simulink model "Waehrungsmodelle"  (R2014a)
settings: Solver=ode1  StartTime=0.0  StopTime=100  FixedStep=1  MaxStep=1  MinStep=1  RelTol=1e-3
(part 2 of 18)

== matlab function Waehrungsmodelle/Währungssystem2/Notenbank/MATLAB Function ==
  data: Gesamtkredite input; LeitzinsOut output; MindestreservesatzOut output; MaximaleNotenbankGeldmengeOut output; Arbeitslosenquote input; Inflation input; Wirtschaftswachtsum input
function [LeitzinsOut, MindestreservesatzOut, MaximaleNotenbankGeldmengeOut] = ...
    Notenbank(Gesamtkredite, Arbeitslosenquote, Inflation, Wirtschaftswachtsum)
%# Submodul zur Berechnung der Notenbankprozesse

% Leitzins der Notenbank => 0.03
persistent Leitzins;

% Mindestreservesatz => 0.01
persistent Mindestreservesatz;    

% Maximale Geldmenge, welche von der Notenbank vergeben werden kann
persistent MaximaleNotenbankGeldmenge;   

% festgelegter Geldmengenwachstum => 0.05
% Dieser Wert ist bei gedeckten Währungssystemen notwendig, da hiermit die
% Geldmenge mit dem Gesamtwert des Deckungswerts mitwachsen kann
Geldmengenwachstum = 0.05;

% gewünschte Inflation => 0.02
Inflationsziel = 0.02;

% Inflationstoleranz => 0.02
Inflationstoleranz = 0.02;

% Arbeitslosentoleranzquote => 0.08
Arbeitslosentoleranzquote = 0.08;

% Änderung des Leitzins
Leitzinsaenderung = 0;

    if isempty(Leitzins)
       Leitzins = 0.03;
    end  
    if isempty(Mindestreservesatz)
       Mindestreservesatz = 0.01;
    end  
    if isempty(MaximaleNotenbankGeldmenge)
       MaximaleNotenbankGeldmenge =  1000;
    end       
    
    % Pürfen, ob ein erlaubter Geldmengenwachstum sinnvoll ist
    if Gesamtkredite > MaximaleNotenbankGeldmenge * 0.9
        MaximaleNotenbankGeldmenge = MaximaleNotenbankGeldmenge * (1 + Geldmengenwachstum);
    end
    
    % Wenn das Wirtschaftswachtsum zu gering ist, wird der Leitzins gesenkt
    if Wirtschaftswachtsum < Leitzins
        Leitzinsaenderung = -0.001;
    else
        Leitzinsaenderung = 0.001;
    end
    
    % Wenn die Arbeitslosigkeit unter der Arbeitslosentoleranzquote ist, wird kann der Leitzins erhöht
    % sonst wird der Leitzins in Abhängigkeit der Arbeitslosenquote gesenkt
    Leitzinsaenderung = Leitzinsaenderung + max(-0.01,0.1 * (Arbeitslosentoleranzquote - Arbeitslosenquote) + 0.001);
    
    % Inflation mit dem Leitzins an die Zielinflation anpassen
    Leitzinsaenderung = Leitzinsaenderung + 0.01 * (Inflation - (Inflationsziel + Inflationstoleranz));
        
    if Leitzins < 0.01 && Leitzinsaenderung < -0.001
        Leitzins = Leitzins - 0.001;
    else        
        Leitzins = Leitzins + Leitzinsaenderung;
    end
    
LeitzinsOut = Leitzins;
MindestreservesatzOut = Mindestreservesatz;
MaximaleNotenbankGeldmengeOut = MaximaleNotenbankGeldmenge;

== matlab function Waehrungsmodelle/Währungssystem2/Unternehmen/MATLAB Function ==
  data: Inflation output; Rohstoffbedarf output; ArbeitsplaetzeUnternehmen output; GueterangebotInland output; ArbeitslohnOut output; Erwerbsfaehige input; BenoetigterArbeitsbedarfUnternehmen output; GueterpreisOut output; NeueKreditvergabeUnternehmen input; KreditrueckzahlungUnternehmen input; SteuernUnternehmen output; RessourcenAbgabeSteuer output; KreditbedarfInland output; Rohstoffe input; GueterkonsumInland input; GueterkonsumAusland input; RessourcenAbgabeSteuersatz input; KreditZinssatzInland input; KreditZinssatzAusland input; Steuersatz input; KreditbedarfAusland output; TechnischeVerbesserungRationalitaetOut output; TechnischeVerbesserungRessourcenOut output; Wirtschaftswachstum output; GueterangebotAusland output; NeueKreditvergabeUnternehmenAusland input; KreditrueckzahlungUnternehmenAusland input
function [Inflation, Rohstoffbedarf, ArbeitsplaetzeUnternehmen, GueterangebotInland, ...
            ArbeitslohnOut, BenoetigterArbeitsbedarfUnternehmen, GueterpreisOut, ...
            SteuernUnternehmen, RessourcenAbgabeSteuer, KreditbedarfInland, KreditbedarfAusland,  ...
            TechnischeVerbesserungRationalitaetOut, TechnischeVerbesserungRessourcenOut, ...
            Wirtschaftswachstum, GueterangebotAusland] = ...
   Unternehmen(Erwerbsfaehige, NeueKreditvergabeUnternehmen, KreditrueckzahlungUnternehmen, ...
            Rohstoffe, GueterkonsumInland, GueterkonsumAusland, RessourcenAbgabeSteuersatz, ...
            KreditZinssatzInland, KreditZinssatzAusland, Steuersatz, ...
            NeueKreditvergabeUnternehmenAusland, KreditrueckzahlungUnternehmenAusland)
        %# Submodul zur Berechnung der Prozessabläufe in Beziehung mit den Unternehmen

% Arbeitslohn
persistent Arbeitslohn;          
        
% Geldbestand
persistent Geldbestand;  
        
% Rohstoffbestand
persistent Rohstoffbestand;   
        
% produzierter Güterbestand
persistent Gueterbestand;   

% Preis zu dem das produzierte Gut verkauft wird
persistent Gueterpreis;  

% technische Effizienzverbesserung bzgl. der Rationalisierung der Arbeiter
persistent TechnischeVerbesserungRationalitaet;   

% technische Effizienzverbesserung bzgl. der Ressourcenverwendung
persistent TechnischeVerbesserungRessourcen;

% Letzte Anzahl an Mitarbeitern
persistent LetzteArbeitsplaetzeUnternehmen;

% Umsatz / Einnahmen
persistent Einnahmen;

% alte Inflation
persistent InflationAlt;

% Geldbestand Initial
if isempty(Geldbestand)
   Geldbestand = 50;
end
% Arbeitslohn Initial
if isempty(Arbeitslohn)
   Arbeitslohn = 3.5;
end
% Rohstoffbestand Initial
if isempty(Rohstoffbestand)
   Rohstoffbestand = 50;
end
% Güterbestand Initial
if isempty(Gueterbestand)
   Gueterbestand = 50;
end 
% Güterpreis Initial
if isempty(Gueterpreis)
   Gueterpreis = 3;
end 
% technische Effizienzverbesserung Rationalisierung Initial
if isempty(TechnischeVerbesserungRessourcen)
   TechnischeVerbesserungRessourcen = 1;
end
% technische Effizienzverbesserung Ressourcenverwendung Initial
if isempty(TechnischeVerbesserungRationalitaet)
   TechnischeVerbesserungRationalitaet = 1;
end
% Umsatz / Einnahmen Initial
if isempty(Einnahmen)
   Einnahmen = 0;
end
if isempty(InflationAlt)
   InflationAlt = 0;
end
% Letzte Anzahl an Mitarbeitern
if isempty(LetzteArbeitsplaetzeUnternehmen)
   LetzteArbeitsplaetzeUnternehmen = 20;
end

% Steigerung der Effizienzen bei technischen Verbesserungen Rationalität
EffizienzsteigerungRationalitaet = 0.04;
% Steigerung der Effizienzen bei technischen Verbesserungen Ressourcen
EffizienzsteigerungRessourcen = 0.02;
% Kosten einer technischen Verbesserung
Verbesserungskosten = 20;
% Steigerung der Kosten bei technischen Verbesserungen
Verbesserungskostensteigerung = 0.2;
% Angestrebter Gewinn
AngestrebterGewinn = 0.1;
% Maximale Preissteierung
MaximalePreissteierung = 0.15;
% Speicherung des letzten Güterpreises
AlterGueterpreis = Gueterpreis;
% Speicherung der letzten Einnahmen
AlteEinnahmen = Einnahmen;
% Menge produzierter Güter pro Mitarbeiter
ProduzierteMengeProMitarbeiter = 1.2;
% Gehaltssteigerung bei Rationalisierung und Gewinn
Gehaltssteigerung = 0.05;
% angestrebter Gütervorrat
GewuenschterGuetervorrat = 200;
% angestrebter Geldbestand
GewuenschterGeldbestand = 200;
% Maximale Entlassungen in Prozent
MaximaleEntlassungsrate = 0.2;

    % vergebene Kredite
    Geldbestand = Geldbestand + NeueKreditvergabeUnternehmen + NeueKreditvergabeUnternehmenAusland;
    % Ratenzahlung der aktuelen Kredite
    Geldbestand = Geldbestand - KreditrueckzahlungUnternehmen + KreditrueckzahlungUnternehmenAusland;

    % Berechnung der Ressourcenangabe
    RessourcenAbgabeSteuer = max(0, RessourcenAbgabeSteuersatz) * Rohstoffe;
    Rohstoffbestand = Rohstoffbestand + Rohstoffe;
    
    % In- und Auslandskonsum summieren
    Gueterkonsum = GueterkonsumInland + GueterkonsumAusland;
    
    % Güterbestand nach den von abgenommene Güter der Haushalten bei 
    % der letzten Zeiteinheit 
    Gueterbestand = Gueterbestand - Gueterkonsum;
    
    % Berechnung der Einnahmen
    Einnahmen = Gueterkonsum * Gueterpreis;
    
    % Berechnung der zu produzierenden Gütermenge (mit 30% Reserve) wenn
    % der Bestand kleiner als 200% des Güterkonsums in einer Zeiteinheit
    % Dabei werden 50 Güter als Reserve in Bestand vorgehalten
    if Gueterbestand < Gueterkonsum * 2
        ProduzierndeGuetermenge = max(5, (1.3 * Gueterkonsum) - (Gueterbestand - GewuenschterGuetervorrat));  
    elseif Gueterbestand < GewuenschterGuetervorrat
        ProduzierndeGuetermenge = Gueterkonsum + (GewuenschterGuetervorrat - Gueterbestand);
    else
       ProduzierndeGuetermenge = max(5, Gueterkonsum / 2);      
    end
    
    % Produktiongüter pro Mitarbeiter in Abhängigkeit
    % der technischen Verbesserung (normal 2 Güter pro Mitarbeiter)
    ProduktionProMitarbeiter = (((1 + EffizienzsteigerungRationalitaet) ^ TechnischeVerbesserungRationalitaet) * ProduzierteMengeProMitarbeiter);
    
    % Ressourcen pro hergestelltes Gut in Abhängigkeit
    % der technischen Verbesserung (normal 1 Güter pro Ressource)    
    RessourcenProGut = (1 / (1 + EffizienzsteigerungRessourcen)) ^ TechnischeVerbesserungRessourcen;
    
    % Zur Berechnung der benötigten Arbeitskraft im nächsten Zeitabschnitt´
    BenoetigterArbeitsbedarfUnternehmen = floor(ProduzierndeGuetermenge / ProduktionProMitarbeiter) + 1;           
    
    % Berechnung der maximal erstellbaren Gütermenge
    MaximaleGueterherstellungErwerbstaetige = Erwerbsfaehige * ProduktionProMitarbeiter;
    MaximaleGueterherstellungRohstoffe = Rohstoffbestand / RessourcenProGut;    
    % Entweder ist die Herstellung durch die Nachfrage, den Arbeitskreaften
    % oder den Ressourcen beschränkt
    Gueterherstellung = min(ProduzierndeGuetermenge, min(MaximaleGueterherstellungErwerbstaetige, MaximaleGueterherstellungRohstoffe));
    Gueterherstellung = max(Gueterherstellung, 0);  
    
    % Berechnung der aktuellen Arbeitsplätze
    ArbeitsplaetzeUnternehmen = floor(Gueterherstellung / ProduktionProMitarbeiter)+1;
    
    % Berechnung der maximalen möglichen Entlassungen
    % Es können max. 20% der Mitarbeiter entlassen werden    
    if ArbeitsplaetzeUnternehmen < LetzteArbeitsplaetzeUnternehmen * (1-MaximaleEntlassungsrate)
        ArbeitsplaetzeUnternehmen = LetzteArbeitsplaetzeUnternehmen * (1-MaximaleEntlassungsrate);
        MaximaleGueterherstellungErwerbstaetige = ArbeitsplaetzeUnternehmen * ProduktionProMitarbeiter;
        Gueterherstellung = min(ProduzierndeGuetermenge, min(MaximaleGueterherstellungErwerbstaetige, MaximaleGueterherstellungRohstoffe));        
    end
    
    % Vergleich der Arbeitsnachfrage mit dem Arbeitsangebot
    ArbeitsangebotsNachfrageQuotient = ArbeitsplaetzeUnternehmen / Erwerbsfaehige;
    % Anpassung der Arbeitslöhne an das Angebot und die Nachfrage der
    % Arbeitsplaetze - max 3% Lohnsenkung oder Lohnsteigerung
    ArbeitsangebotsNachfrageQuotient= max(0.94,min(1.04,(ArbeitsangebotsNachfrageQuotient + 0.3)));
    Arbeitslohn = Arbeitslohn * ArbeitsangebotsNachfrageQuotient;
    
    % Berechnung der aktuell verbrauchten Ressourcen
    Rohstoffbestand = Rohstoffbestand - (floor(Gueterherstellung * RessourcenProGut)+1);
    
    % hergestellte Gütermenge
    Gueterbestand = Gueterbestand + Gueterherstellung;
    
    % Als Export-Angebot werden 30% der Güter vorgesehen
    GueterangebotAusland = Gueterbestand * 0.3;
    GueterangebotInland = Gueterbestand - GueterangebotAusland;          
    
    % Berechnung der Gehälter
    Gehaelter = ArbeitsplaetzeUnternehmen * Arbeitslohn;
    
    % Vorteil einer Investitionen-Rationalität berechnen
    InvestPruefungProduktionProMitarbeiter = (((1 + EffizienzsteigerungRationalitaet) ^ (TechnischeVerbesserungRationalitaet + 1)) * 2);
    InvestPruefungArbeitsplaetzeUnternehmen = floor(Gueterherstellung / InvestPruefungProduktionProMitarbeiter)+1;    
    InvesteinsparungRationalitaet = Arbeitslohn * (ArbeitsplaetzeUnternehmen - InvestPruefungArbeitsplaetzeUnternehmen);
    % Vorteil einer Investitionen-Ressourceneffizienz berechnen
    InvestPruefungRessourcenProGut = (1 / (1 + EffizienzsteigerungRessourcen)) ^ (TechnischeVerbesserungRessourcen + 1);
    InvestPruefungRessourcenbedarf = floor(Gueterherstellung * InvestPruefungRessourcenProGut)+1;    
    InvesteinsparungRessourcenbedarf = RessourcenAbgabeSteuersatz * ((Gueterherstellung * RessourcenProGut) - InvestPruefungRessourcenbedarf);    
    
    % Kosten für die nächste Investitionsstufe berechnen
    InvestkostenRationalitaet = Verbesserungskosten * (1 + Verbesserungskostensteigerung) ^ (TechnischeVerbesserungRationalitaet + 1);
    InvestkostenRessourcenEffizienz = Verbesserungskosten * (1 + Verbesserungskostensteigerung) ^ (TechnischeVerbesserungRessourcen + 1);
    
    % Prüfen, ob und welche Investition mehr Sinn macht
    % Das vorhandene Geld muss dabei doppelt so hoch sein, damit nicht mit
    % dem letzten Geld Investitionen durchgeführt werden
    Investition = 0;
    if (InvesteinsparungRationalitaet > InvesteinsparungRessourcenbedarf) && Geldbestand > InvestkostenRationalitaet*2 && InvesteinsparungRationalitaet > 0
        % Verbesserung Rationalität
        TechnischeVerbesserungRationalitaet = TechnischeVerbesserungRationalitaet + 1;
        Investition = InvestkostenRationalitaet;
        % Anstieg des Arbeitslohn auf Grund der Rationalitätsgewinne 
        Arbeitslohn = Arbeitslohn * (1 + Gehaltssteigerung);
    elseif Geldbestand > InvestkostenRessourcenEffizienz*2 && InvesteinsparungRessourcenbedarf > 0;
        % Verbesserung Ressourceneffizienz
        TechnischeVerbesserungRessourcen = TechnischeVerbesserungRessourcen + 1;
        Investition = InvestkostenRessourcenEffizienz;
    end
    
    % Ausgaben berechnen
    Ausgaben = RessourcenAbgabeSteuer + Gehaelter;
    
    % Der Preis der produzierten Warten richtet sich NICHT nach der Nachfrage 
    % und dem Angebot, sondern nach den Herrstellungskosten und dem 
    % angestrebten Gewinn. Welches ist der niedrigste Preis, damit das 
    % Unternehmen den angestrebten Gewinn erwirtschaftet und Investieren
    % kann
    Herstellkosten = Ausgaben / Gueterherstellung;
    % Es gibt eine maximale Preisteigerung welche durchgesetzt werden kann
    MaximalerGueterpreis = (1 + MaximalePreissteierung) * Gueterpreis;
    Gueterpreis = min(MaximalerGueterpreis, Herstellkosten * (1 + AngestrebterGewinn));   
    
    % Berechnung der Inflation
    Inflation = (InflationAlt + (Gueterpreis / AlterGueterpreis) - 1) / 2;
    InflationAlt = Inflation;
                
    % Gewinnberechnung
    Gewinn = Einnahmen - Ausgaben;            
    
    if Gewinn > 0
        % Anstieg des Arbeitslohn auf Grund der Gewinnsteigerung               
        Arbeitslohn = Arbeitslohn * (1 + Gehaltssteigerung);  
        
        % Steuerberechnung vom Gewinn
        SteuernUnternehmen = Gewinn * Steuersatz;
    else
        SteuernUnternehmen = 0;
    end

    Geldbestand = Geldbestand + Gewinn - (SteuernUnternehmen + Investition);
       
    % Wenn notwendig, neuen Kredit beantragen
    if Geldbestand < GewuenschterGeldbestand                
        % Kreditbedarf berechnen
        Kreditbedarf = GewuenschterGeldbestand - Geldbestand;
    else 
        Kreditbedarf = 0;
    end         
    
    % Kreditbedarf auf In- und Ausland aufteilen
    % Der Kredit mit dem geringeren Zinssatz wird bevorzugt und 70%
    % verwendet. Der teurere Kredit wird mit 30% verwendet.
    if KreditZinssatzInland <= KreditZinssatzAusland
        KreditbedarfInland = Kreditbedarf * 0.7;
        KreditbedarfAusland = Kreditbedarf * 0.3;
    else
        KreditbedarfAusland = Kreditbedarf * 0.7;
        KreditbedarfInland = Kreditbedarf * 0.3;        
    end

    % Berechnung der benötigten Ressourcen im nächsten Zeitabschnitt    
    Rohstoffbedarf = max(0, floor(Gueterherstellung * RessourcenProGut) + GewuenschterGuetervorrat - Rohstoffbestand);            
    
    % Auf Grund der Angebots-/Nachfragesituation kann der Güterpreis nicht
    % unter dem Arbeitslohn sein
    Gueterpreis = min(Gueterpreis, Arbeitslohn);
    % Wenn kein Konsum stattgefunden hat sinkt der Preis
    if GueterkonsumInland == 0
        Gueterpreis = Gueterpreis * (1-MaximalePreissteierung);
    end
    
    
    Wirtschaftswachstum = (Einnahmen / AlteEinnahmen) - 1;
    
    ArbeitslohnOut = Arbeitslohn;
    GueterpreisOut = Gueterpreis;
    TechnischeVerbesserungRationalitaetOut = TechnischeVerbesserungRationalitaet;
    TechnischeVerbesserungRessourcenOut = TechnischeVerbesserungRessourcen;
    LetzteArbeitsplaetzeUnternehmen = ArbeitsplaetzeUnternehmen;

== matlab function Waehrungsmodelle/Fließendes Währungssystem/Staat/MATLAB Function ==
  data: KreditvergabeNeuStaat input; Kreditrueckzahlung input; FinanzbedarfArbeitslosigkeit input; Dienstleistungsqualitaet input; Kreditbedarf output; SteuernBanken input; SteuernUnternehmen input; Rohstoffabgabe input; FinanzierungOeffentlicheDienstleistungen output; GeldbestandStaat output; SteuersatzOut output; RessourcenAbgabesatzOut output; Umweltqualitaet input; Liquiditaetsabgabe input
function [Kreditbedarf, FinanzierungOeffentlicheDienstleistungen, GeldbestandStaat, ...
            SteuersatzOut, RessourcenAbgabesatzOut] = ...
    Staat(KreditvergabeNeuStaat, Kreditrueckzahlung, FinanzbedarfArbeitslosigkeit, ...
            Dienstleistungsqualitaet, SteuernBanken, SteuernUnternehmen, Rohstoffabgabe, Umweltqualitaet, Liquiditaetsabgabe)
%# Submodul zur Berechnung der Staatsprozesse

    % Geldbestand
    persistent Geldbestand;    

    % letzte Finanzierung
    persistent LetzteFinanzierung;
    
    % Steuersatz in Prozent
    persistent Steuersatz;  
    
    % Ressourcenabgabesatz
    persistent RessourcenAbgabesatz;
    
    % Geldbestand
    if isempty(Geldbestand)
       Geldbestand = 100;
    end 
    % letzte Finanzierung
    if isempty(LetzteFinanzierung)
       LetzteFinanzierung = 30;
    end 
    % Steuersatz in Prozent
    if isempty(Steuersatz)
       Steuersatz = 0.4;
    end     
    % Ressourcenabgabesatz
    if isempty(RessourcenAbgabesatz)
       RessourcenAbgabesatz = 0.6;
    end       
    
    % Maximaler Steuersatz
    MaximalerSteuersatz = 0.6;
    
    % Steuereinkommen
    Steuereinkommen = SteuernBanken + SteuernUnternehmen + Rohstoffabgabe + Liquiditaetsabgabe;
    
    % Abzug Kosten für Arbeitslose und Kreditrueckzahlung
    Steuereinkommen = Steuereinkommen  - (Kreditrueckzahlung + FinanzbedarfArbeitslosigkeit);
    
    % Aktuallisierung des Geldbestands
    Geldbestand = Geldbestand + Steuereinkommen + KreditvergabeNeuStaat;
    
    % Prüfen des Finanzierungsbedarfs
    if Dienstleistungsqualitaet > 0.9
        Finanzierungsbedarf = LetzteFinanzierung;        
    elseif Dienstleistungsqualitaet < 0.4
        Finanzierungsbedarf = LetzteFinanzierung * 1.05+5;   
    elseif Dienstleistungsqualitaet < 0.7
        Finanzierungsbedarf = LetzteFinanzierung * 1.02;           
    else
        Finanzierungsbedarf = LetzteFinanzierung * 1.01;        
    end                 

    Kreditbedarf = 0;
    % Prüfen ob der Steuersatz geändert werden sollte
    if Geldbestand > 150
        Steuersatz = max(0, Steuersatz - 0.01);   
    else
        Steuersatz = min(MaximalerSteuersatz, Steuersatz + 0.01);        
        Finanzierungsbedarf = LetzteFinanzierung * 0.9;
        % Wenn wenig Geld vorhanden ist, Kredit beantragen
        Kreditbedarf = (FinanzbedarfArbeitslosigkeit + Finanzierungsbedarf + 10) - Steuereinkommen;  
    end                
    
    FinanzierungOeffentlicheDienstleistungen = Finanzierungsbedarf;
    
    % Abgaben der Ressourcenabgabe berechnen
    if (Umweltqualitaet < 0.5)
        RessourcenAbgabesatz = RessourcenAbgabesatz + 0.02;    
    elseif (Umweltqualitaet < 0.7)
        RessourcenAbgabesatz = RessourcenAbgabesatz + 0.01;
    elseif (Umweltqualitaet > 0.9)
        RessourcenAbgabesatz = RessourcenAbgabesatz - 0.01;
    end
    
    % Kosten vom Geldbestand abziehen
    Geldbestand  = Geldbestand - FinanzierungOeffentlicheDienstleistungen;
       
    % Speichern der Werte
    LetzteFinanzierung = FinanzierungOeffentlicheDienstleistungen;
    SteuersatzOut = Steuersatz;
    GeldbestandStaat = Geldbestand;
    RessourcenAbgabesatzOut = RessourcenAbgabesatz;

== matlab function Waehrungsmodelle/Währungssystem5/Banken/MATLAB Function ==
  data: EinlagenAenderungHaushalte input; KreditbedarfHaushalte input; KreditbedarfUnternehmen input; KreditbedarfHaushalteAusland input; KreditbedarfUnternehmenAusland input; KreditbedarfStaat input; Steuersatz input; Leitzins input; Mindestreservesatz input; MaximaleNotenbankGeldmenge input; KontoHaushalteOut output; KrediteHaushalteOut output; KrediteUnternehmenOut output; KrediteStaatOut output; KreditvergabeHaushalte output; KreditvergabeUnternehmen output; KreditvergabeStaat output; KreditrueckzahlungHaushalte output; KreditrueckzahlungUnternehmen output; KreditrueckzahlungStaat output; BankgewinnNachSteuern output; BankenSteuern output; BankKontostand output; Bankenzinssatz output; KrediteUnternehmenAuslandOut output; KreditrueckzahlungUnternehmenAusland output; KreditvergabeUnternehmenAusland output; KrediteHaushalteAuslandOut output; KreditrueckzahlungHaushalteAusland output; KreditvergabeHaushalteAusland output
function [KontoHaushalteOut, KrediteHaushalteOut, KrediteUnternehmenOut, KrediteStaatOut, ... 
            KreditvergabeHaushalte, KreditvergabeUnternehmen, KreditvergabeStaat, ...
            KreditrueckzahlungHaushalte, KreditrueckzahlungUnternehmen, KreditrueckzahlungStaat, ...
            BankgewinnNachSteuern, BankenSteuern, BankKontostand, Bankenzinssatz, ...
            KrediteUnternehmenAuslandOut, KreditrueckzahlungUnternehmenAusland, KreditvergabeUnternehmenAusland, ...
            KrediteHaushalteAuslandOut, KreditrueckzahlungHaushalteAusland, KreditvergabeHaushalteAusland] = ...
    Banken(EinlagenAenderungHaushalte, KreditbedarfHaushalte, KreditbedarfUnternehmen, ...
            KreditbedarfHaushalteAusland, KreditbedarfUnternehmenAusland, KreditbedarfStaat, ...
            Steuersatz, Leitzins, Mindestreservesatz, MaximaleNotenbankGeldmenge)
% Submodell Banken zur Berechnung der Geld-Prozesse zwischen 
% Banken und Haushalten

% ANMERKUNG:
% Warum gibt es auf der einen Seite Kredite und Guthaben der Haushalte?
% Der überwigende Teil der Geldes MUSS den Haushalten gehören, da diese
% die Unternehmen und Banken besitzen. Ich vermute, dass es in einen
% demokratischen Staat nicht möglich ist, dass der Staat mehr Geld als 
% die Bevölkerung besitzt.
% Die ungleiche Geldverteilung ist dafür verantwortlich, dass die Haushalte
% auf der einen Seite Spareinlagen und Kredite haben. Ohne Spareinlagen wäre
% es aktuell nicht möglich Kredite überhaupt zu vergeben.

% Der Zinsspread ist die Prozentuale-Differenz der Zinsweitergabe bei
% Krediten und Anlagen
persistent Zinsspread;

% interner Zinssatz
persistent InternerZinssatz;

% aktuelle Kredithöhe der Unternehmen
persistent KrediteUnternehmen;

% aktuelle Kredithöhe des Staats
persistent KrediteStaat;

% aktuelle Kredithöhe der Haushalte
persistent KrediteHaushalte;

% aktuelle Kredithöhe der Unternehmen im Ausland
persistent KrediteUnternehmenAusland;

% aktuelle Kredithöhe der Haushalte im Ausland
persistent KrediteHaushalteAusland;

% aktueller Kontostand der Haushalte
persistent KontoHaushalte;

% Rückzahlungsdauer des Kredits
persistent Kreditrueckzahlungsdauer;

% Vermnögen der Bank aus den Gewinnen
persistent KontoBank;

    % Zinsspread 1%
    if isempty(Zinsspread)
       Zinsspread = 0.01;
    end 
    
    % interner Zinssatz auf den Leitzins festlegen
    if isempty(InternerZinssatz)
       InternerZinssatz = Leitzins;
    end     
    
    % Rückzahlungsdauer 15 Zeiteinheiten
    if isempty(Kreditrueckzahlungsdauer)
       Kreditrueckzahlungsdauer = 15;
    end     
   
    if isempty(KontoBank)
       KontoBank = 400;
    end   
    if isempty(KontoHaushalte)
       KontoHaushalte = 0;
    end   
    if isempty(KrediteHaushalte)
       KrediteHaushalte = 200;
    end     
    if isempty(KrediteUnternehmen)
       KrediteUnternehmen = 200;
    end 
    if isempty(KrediteStaat)
       KrediteStaat = 200;
    end     
    if isempty(KrediteUnternehmenAusland)
       KrediteUnternehmenAusland = 200;
    end     
    if isempty(KrediteHaushalteAusland)
       KrediteHaushalteAusland = 200;
    end   
    
    % Habenzinsen berechnen
    HabenZinsen = KontoHaushalte * (InternerZinssatz - Zinsspread);
    KontoHaushalte = KontoHaushalte + HabenZinsen;
    
    % Ein- / Auszahlung
    KontoHaushalte = KontoHaushalte + EinlagenAenderungHaushalte;    
      
    % Maximale Kreditvergabe anhand des Mindestreservesatzes und der 
    % Spareinlagen der Haushalte
    MaximaleKreditvergabe = KontoHaushalte * (1 / Mindestreservesatz); 

    % Maximale Geldmenge, welche von der Notenbank zur Verfügung gestellt wird
    % Prüfung anhand der Maximalen Kreditvergabe, da Guthaben = Kredit    
    MaximaleKreditvergabe = max(MaximaleNotenbankGeldmenge, MaximaleKreditvergabe);
    
    Gesamtkredit = KrediteHaushalte + KrediteUnternehmen + KrediteStaat;
    MaximaleKreditvergabe = MaximaleKreditvergabe - Gesamtkredit;

    % Wenn genug Geld auf dem Konto ist, so wird ein prozenualer Anteil mit
    % dem neuen Kreditbedarf verrechnet ==> 10 %    
    if KontoHaushalte > KreditbedarfHaushalte && KreditbedarfHaushalte > 0
       AusgleichbarerGeldBedarf = KreditbedarfHaushalte * 0.1;
       KontoHaushalte = KontoHaushalte - AusgleichbarerGeldBedarf;
       KreditbedarfHaushalte = KreditbedarfHaushalte - AusgleichbarerGeldBedarf;
    end         

    % Kreditberechnung für Haushalte      
    [KrediteHaushalte, KreditvergabeHaushalte, KreditrueckzahlungHaushalte, ...
                        SollZinsenHaushalte, MaximaleKreditvergabe] = ...
        Kreditberechnung(KrediteHaushalte, KreditbedarfHaushalte, MaximaleKreditvergabe, ...
                        InternerZinssatz, Zinsspread, Kreditrueckzahlungsdauer);                    
    
    % Kreditberechnung für Staat   
    [KrediteStaat, KreditvergabeStaat, KreditrueckzahlungStaat, SollZinsenStaat, ...
                        MaximaleKreditvergabe] = ...
        Kreditberechnung(KrediteStaat, KreditbedarfStaat, MaximaleKreditvergabe, ...
                        InternerZinssatz, Zinsspread, Kreditrueckzahlungsdauer);                    

    % Kreditberechnung für Unternehmen   
    [KrediteUnternehmen, KreditvergabeUnternehmen, KreditrueckzahlungUnternehmen, ...
                        SollZinsenUnternehmen, MaximaleKreditvergabe] = ...
        Kreditberechnung(KrediteUnternehmen, KreditbedarfUnternehmen, MaximaleKreditvergabe, ...
                        InternerZinssatz, Zinsspread, Kreditrueckzahlungsdauer);

    % Kreditberechnung für Haushalte im Ausland
    [KrediteHaushalteAusland, KreditvergabeHaushalteAusland, KreditrueckzahlungHaushalteAusland, ...
                        SollZinsenHaushalteAusland, MaximaleKreditvergabe] = ...
        Kreditberechnung(KrediteHaushalteAusland, KreditbedarfHaushalteAusland, MaximaleKreditvergabe, ...
                        InternerZinssatz, Zinsspread, Kreditrueckzahlungsdauer);                                        

    % Kreditberechnung für Unternehmen im Ausland
    [KrediteUnternehmenAusland, KreditvergabeUnternehmenAusland, KreditrueckzahlungUnternehmenAusland, ...
                        SollZinsenUnternehmenAusland, MaximaleKreditvergabe] = ...
        Kreditberechnung(KrediteUnternehmenAusland, KreditbedarfUnternehmenAusland, MaximaleKreditvergabe, ...
                        InternerZinssatz, Zinsspread, Kreditrueckzahlungsdauer);                    
                    
    % Berechnung der Notenbankkredite
    NotenbankKredite = (KrediteHaushalte + KrediteUnternehmen + KrediteStaat + ...
                    KrediteHaushalteAusland + KrediteUnternehmenAusland) - (KontoBank + KontoHaushalte);
    NotenbankKredite = max(NotenbankKredite, 0);
    NotenbankZinsen = NotenbankKredite * Leitzins;
    KontoBank = KontoBank - NotenbankZinsen;   
    
    % Gewinnberechnung der Bank
    SollZinsen = SollZinsenHaushalte + SollZinsenStaat + SollZinsenUnternehmen ...
                + SollZinsenHaushalteAusland + SollZinsenUnternehmenAusland;
    Bankgewinn = SollZinsen - HabenZinsen;
    
    % Steuerberechnung der Bank
    BankenSteuern = max(Bankgewinn * Steuersatz, 0);
    BankgewinnNachSteuern = Bankgewinn - BankenSteuern;
    
    % Kontostand der Bank berechnen
    KontoBank = KontoBank + Bankgewinn - BankenSteuern;
    
    % Zinssätze anpassen (Zinsänderung anpassen y = -0.00005x + 0.0025;
    Zinsaenderung = -0.00005 * BankgewinnNachSteuern + 0.001;
    InternerZinssatz = InternerZinssatz + Zinsaenderung;
    
    KrediteStaatOut = KrediteStaat;
    KrediteUnternehmenOut = KrediteUnternehmen;
    KrediteHaushalteOut = KrediteHaushalte;
    KrediteUnternehmenAuslandOut = KrediteUnternehmenAusland;
    KrediteHaushalteAuslandOut = KrediteHaushalteAusland;    
    KontoHaushalteOut = KontoHaushalte;    
    BankKontostand = KontoBank;
    Bankenzinssatz = InternerZinssatz;

== matlab function Waehrungsmodelle/Vollgeld Währungssystem/Umwelt/Umwelt ==
  data: Ressourcenbedarf input; AbgebauteRessourcen output; VorhandeneRessourcenOut output; Umweltqualitaet output
function [AbgebauteRessourcen, VorhandeneRessourcenOut, Umweltqualitaet] = Umwelt(Ressourcenbedarf)
%# Submodell zum Prozessablauf der Umwelt und der Ressourcen


% Vorhandene Ressourcen
persistent VorhandeneRessourcen;

% Initiale Ressourcen
InitialeRessourcen = 2500;
% Maximale Abbaurate
MaximaleAbbaurate = 0.1;
% Ressourcenregenerationsrate
Ressourcenregenerationsrate = 0.02;
    
% Vorhandene Ressourcen Initial
if isempty(VorhandeneRessourcen)
   VorhandeneRessourcen = InitialeRessourcen;
end

    % Berechnung der maximal abbaubaren Ressourcen
    MaximalAbbaubareRessourcen = VorhandeneRessourcen * MaximaleAbbaurate;
    
    % abgebaute Ressourcen
    AbgebauteRessourcen = min(MaximalAbbaubareRessourcen, Ressourcenbedarf);       
    VorhandeneRessourcen = VorhandeneRessourcen - AbgebauteRessourcen;
    
    % Ressourcen Regeneration
    VorhandeneRessourcen = VorhandeneRessourcen * (1  + Ressourcenregenerationsrate);    
    
    % Umweltqualitaet berechnen
    Umweltqualitaet = max(min(VorhandeneRessourcen / InitialeRessourcen, 1), 0);
        
    VorhandeneRessourcenOut = VorhandeneRessourcen;

== matlab function Waehrungsmodelle/Vollgeld Währungssystem/Öffentliche Dienstleistungen/MATLAB Function ==
  data: Finanzierung input; ArbeitsplaetzeDienstleistung output; Erwerbsfaehige input; Arbeitslohn input; Dienstleistungsqualitaet output
function [ArbeitsplaetzeDienstleistung, Dienstleistungsqualitaet] = OeffentlicheDienstleistungen(Finanzierung, Erwerbsfaehige, Arbeitslohn)
%# Submodul zur Berechnung das Öffentliche Dienstleistungsmodell

    persistent Arbeitsplaetze;

    % Anfangsarbeitsplätze
    if isempty(Arbeitsplaetze)
       Arbeitsplaetze = 20;
    end 

    % Da der Arbeitslohn ein Referenzlohn der privaten Unternehmen ist wird
    % dieser angepasst und um 20 % gesenkt
    LohnNiveauOeffentlicherDienst = 0.8;
    Arbeitslohn = Arbeitslohn * LohnNiveauOeffentlicherDienst;
    
    % Es können nicht mehr Arbeitsplätze wie Erwerbsfähige vorhanden sind
    % besetzt werden
    if Erwerbsfaehige < Arbeitsplaetze
        Arbeitsplaetze = Erwerbsfaehige;
    end

    % Existiert nicht genug Geld für die öffentlichen Dientleistungen
    % werden die Arbeitsplätze an die Finanzierung vom Staat angepasst.
    if (Finanzierung < Arbeitsplaetze * Arbeitslohn)
        Arbeitsplaetze = floor(Finanzierung / Arbeitslohn);        
    end          
       
    ArbeitsplaetzeDienstleistung = Arbeitsplaetze;
    
    % Berechnet Dienstleistungsqualitaet mit min:0.2 und max:1
    % indem die Arbeitsplätze der öffentlichen Dienstleistungen durch die
    % gesamten Erwerbstätigen geteilt werden und als Ausgleichfaktor mit drei
    % multipliziert wird. Somit ist es optimal wenn min. 1/3 aller
    % Erwerbsfähigen bei den öffentlichen Dienstleistungen arbeiten
    Dienstleistungsqualitaet = max(0.2, min(1, 3 * Arbeitsplaetze / Erwerbsfaehige));

== matlab function Waehrungsmodelle/Währungssystem3/Notenbank/MATLAB Function ==
  data: Gesamtkredite input; LeitzinsOut output; MindestreservesatzOut output; MaximaleNotenbankGeldmengeOut output; Arbeitslosenquote input; Inflation input; Wirtschaftswachtsum input
function [LeitzinsOut, MindestreservesatzOut, MaximaleNotenbankGeldmengeOut] = ...
    Notenbank(Gesamtkredite, Arbeitslosenquote, Inflation, Wirtschaftswachtsum)
%# Submodul zur Berechnung der Notenbankprozesse

% Leitzins der Notenbank => 0.03
persistent Leitzins;

% Mindestreservesatz => 0.01
persistent Mindestreservesatz;    

% Maximale Geldmenge, welche von der Notenbank vergeben werden kann
persistent MaximaleNotenbankGeldmenge;   

% festgelegter Geldmengenwachstum => 0.05
% Dieser Wert ist bei gedeckten Währungssystemen notwendig, da hiermit die
% Geldmenge mit dem Gesamtwert des Deckungswerts mitwachsen kann
Geldmengenwachstum = 0.05;

% gewünschte Inflation => 0.02
Inflationsziel = 0.02;

% Inflationstoleranz => 0.02
Inflationstoleranz = 0.02;

% Arbeitslosentoleranzquote => 0.08
Arbeitslosentoleranzquote = 0.08;

% Änderung des Leitzins
Leitzinsaenderung = 0;

    if isempty(Leitzins)
       Leitzins = 0.03;
    end  
    if isempty(Mindestreservesatz)
       Mindestreservesatz = 0.01;
    end  
    if isempty(MaximaleNotenbankGeldmenge)
       MaximaleNotenbankGeldmenge =  1000;
    end       
    
    % Pürfen, ob ein erlaubter Geldmengenwachstum sinnvoll ist
    if Gesamtkredite > MaximaleNotenbankGeldmenge * 0.9
        MaximaleNotenbankGeldmenge = MaximaleNotenbankGeldmenge * (1 + Geldmengenwachstum);
    end
    
    % Wenn das Wirtschaftswachtsum zu gering ist, wird der Leitzins gesenkt
    if Wirtschaftswachtsum < Leitzins
        Leitzinsaenderung = -0.001;
    else
        Leitzinsaenderung = 0.001;
    end
    
    % Wenn die Arbeitslosigkeit unter der Arbeitslosentoleranzquote ist, wird kann der Leitzins erhöht
    % sonst wird der Leitzins in Abhängigkeit der Arbeitslosenquote gesenkt
    Leitzinsaenderung = Leitzinsaenderung + max(-0.01,0.1 * (Arbeitslosentoleranzquote - Arbeitslosenquote) + 0.001); 
    
    % Inflation mit dem Leitzins an die Zielinflation anpassen
    Leitzinsaenderung = Leitzinsaenderung + 0.01 * (Inflation - (Inflationsziel + Inflationstoleranz));
        
    if Leitzins < 0.01 && Leitzinsaenderung < -0.001
        Leitzins = Leitzins - 0.001;
    else        
        Leitzins = Leitzins + Leitzinsaenderung;
    end
    
LeitzinsOut = Leitzins;
MindestreservesatzOut = Mindestreservesatz;
MaximaleNotenbankGeldmengeOut = MaximaleNotenbankGeldmenge;

== matlab function Waehrungsmodelle/Währungssystem3/Unternehmen/MATLAB Function ==
  data: Inflation output; Rohstoffbedarf output; ArbeitsplaetzeUnternehmen output; GueterangebotInland output; ArbeitslohnOut output; Erwerbsfaehige input; BenoetigterArbeitsbedarfUnternehmen output; GueterpreisOut output; NeueKreditvergabeUnternehmen input; KreditrueckzahlungUnternehmen input; SteuernUnternehmen output; RessourcenAbgabeSteuer output; KreditbedarfInland output; Rohstoffe input; GueterkonsumInland input; GueterkonsumAusland input; RessourcenAbgabeSteuersatz input; KreditZinssatzInland input; KreditZinssatzAusland input; Steuersatz input; KreditbedarfAusland output; TechnischeVerbesserungRationalitaetOut output; TechnischeVerbesserungRessourcenOut output; Wirtschaftswachstum output; GueterangebotAusland output; NeueKreditvergabeUnternehmenAusland input; KreditrueckzahlungUnternehmenAusland input
function [Inflation, Rohstoffbedarf, ArbeitsplaetzeUnternehmen, GueterangebotInland, ...
            ArbeitslohnOut, BenoetigterArbeitsbedarfUnternehmen, GueterpreisOut, ...
            SteuernUnternehmen, RessourcenAbgabeSteuer, KreditbedarfInland, KreditbedarfAusland,  ...
            TechnischeVerbesserungRationalitaetOut, TechnischeVerbesserungRessourcenOut, ...
            Wirtschaftswachstum, GueterangebotAusland] = ...
   Unternehmen(Erwerbsfaehige, NeueKreditvergabeUnternehmen, KreditrueckzahlungUnternehmen, ...
            Rohstoffe, GueterkonsumInland, GueterkonsumAusland, RessourcenAbgabeSteuersatz, ...
            KreditZinssatzInland, KreditZinssatzAusland, Steuersatz, ...
            NeueKreditvergabeUnternehmenAusland, KreditrueckzahlungUnternehmenAusland)
        %# Submodul zur Berechnung der Prozessabläufe in Beziehung mit den Unternehmen

% Arbeitslohn
persistent Arbeitslohn;          
        
% Geldbestand
persistent Geldbestand;  
        
% Rohstoffbestand
persistent Rohstoffbestand;   
        
% produzierter Güterbestand
persistent Gueterbestand;   

% Preis zu dem das produzierte Gut verkauft wird
persistent Gueterpreis;  

% technische Effizienzverbesserung bzgl. der Rationalisierung der Arbeiter
persistent TechnischeVerbesserungRationalitaet;   

% technische Effizienzverbesserung bzgl. der Ressourcenverwendung
persistent TechnischeVerbesserungRessourcen;

% Letzte Anzahl an Mitarbeitern
persistent LetzteArbeitsplaetzeUnternehmen;

% Umsatz / Einnahmen
persistent Einnahmen;

% alte Inflation
persistent InflationAlt;

% Geldbestand Initial
if isempty(Geldbestand)
   Geldbestand = 50;
end
% Arbeitslohn Initial
if isempty(Arbeitslohn)
   Arbeitslohn = 3.5;
end
% Rohstoffbestand Initial
if isempty(Rohstoffbestand)
   Rohstoffbestand = 50;
end
% Güterbestand Initial
if isempty(Gueterbestand)
   Gueterbestand = 50;
end 
% Güterpreis Initial
if isempty(Gueterpreis)
   Gueterpreis = 3;
end 
% technische Effizienzverbesserung Rationalisierung Initial
if isempty(TechnischeVerbesserungRessourcen)
   TechnischeVerbesserungRessourcen = 1;
end
% technische Effizienzverbesserung Ressourcenverwendung Initial
if isempty(TechnischeVerbesserungRationalitaet)
   TechnischeVerbesserungRationalitaet = 1;
end
% Umsatz / Einnahmen Initial
if isempty(Einnahmen)
   Einnahmen = 0;
end
if isempty(InflationAlt)
   InflationAlt = 0;
end
% Letzte Anzahl an Mitarbeitern
if isempty(LetzteArbeitsplaetzeUnternehmen)
   LetzteArbeitsplaetzeUnternehmen = 20;
end

% Steigerung der Effizienzen bei technischen Verbesserungen Rationalität
EffizienzsteigerungRationalitaet = 0.04;
% Steigerung der Effizienzen bei technischen Verbesserungen Ressourcen
EffizienzsteigerungRessourcen = 0.02;
% Kosten einer technischen Verbesserung
Verbesserungskosten = 20;
% Steigerung der Kosten bei technischen Verbesserungen
Verbesserungskostensteigerung = 0.2;
% Angestrebter Gewinn
AngestrebterGewinn = 0.1;
% Maximale Preissteierung
MaximalePreissteierung = 0.15;
% Speicherung des letzten Güterpreises
AlterGueterpreis = Gueterpreis;
% Speicherung der letzten Einnahmen
AlteEinnahmen = Einnahmen;
% Menge produzierter Güter pro Mitarbeiter
ProduzierteMengeProMitarbeiter = 1.2;
% Gehaltssteigerung bei Rationalisierung und Gewinn
Gehaltssteigerung = 0.05;
% angestrebter Gütervorrat
GewuenschterGuetervorrat = 200;
% angestrebter Geldbestand
GewuenschterGeldbestand = 200;
% Maximale Entlassungen in Prozent
MaximaleEntlassungsrate = 0.2;

    % vergebene Kredite
    Geldbestand = Geldbestand + NeueKreditvergabeUnternehmen + NeueKreditvergabeUnternehmenAusland;
    % Ratenzahlung der aktuelen Kredite
    Geldbestand = Geldbestand - KreditrueckzahlungUnternehmen + KreditrueckzahlungUnternehmenAusland;

    % Berechnung der Ressourcenangabe
    RessourcenAbgabeSteuer = max(0, RessourcenAbgabeSteuersatz) * Rohstoffe;
    Rohstoffbestand = Rohstoffbestand + Rohstoffe;
    
    % In- und Auslandskonsum summieren
    Gueterkonsum = GueterkonsumInland + GueterkonsumAusland;
    
    % Güterbestand nach den von abgenommene Güter der Haushalten bei 
    % der letzten Zeiteinheit 
    Gueterbestand = Gueterbestand - Gueterkonsum;
    
    % Berechnung der Einnahmen
    Einnahmen = Gueterkonsum * Gueterpreis;
    
    % Berechnung der zu produzierenden Gütermenge (mit 30% Reserve) wenn
    % der Bestand kleiner als 200% des Güterkonsums in einer Zeiteinheit
    % Dabei werden 50 Güter als Reserve in Bestand vorgehalten
    if Gueterbestand < Gueterkonsum * 2
        ProduzierndeGuetermenge = max(5, (1.3 * Gueterkonsum) - (Gueterbestand - GewuenschterGuetervorrat));  
    elseif Gueterbestand < GewuenschterGuetervorrat
        ProduzierndeGuetermenge = Gueterkonsum + (GewuenschterGuetervorrat - Gueterbestand);
    else
       ProduzierndeGuetermenge = max(5, Gueterkonsum / 2);      
    end
    
    % Produktiongüter pro Mitarbeiter in Abhängigkeit
    % der technischen Verbesserung (normal 2 Güter pro Mitarbeiter)
    ProduktionProMitarbeiter = (((1 + EffizienzsteigerungRationalitaet) ^ TechnischeVerbesserungRationalitaet) * ProduzierteMengeProMitarbeiter);
    
    % Ressourcen pro hergestelltes Gut in Abhängigkeit
    % der technischen Verbesserung (normal 1 Güter pro Ressource)    
    RessourcenProGut = (1 / (1 + EffizienzsteigerungRessourcen)) ^ TechnischeVerbesserungRessourcen;
    
    % Zur Berechnung der benötigten Arbeitskraft im nächsten Zeitabschnitt´
    BenoetigterArbeitsbedarfUnternehmen = floor(ProduzierndeGuetermenge / ProduktionProMitarbeiter) + 1;           
    
    % Berechnung der maximal erstellbaren Gütermenge
    MaximaleGueterherstellungErwerbstaetige = Erwerbsfaehige * ProduktionProMitarbeiter;
    MaximaleGueterherstellungRohstoffe = Rohstoffbestand / RessourcenProGut;    
    % Entweder ist die Herstellung durch die Nachfrage, den Arbeitskreaften
    % oder den Ressourcen beschränkt
    Gueterherstellung = min(ProduzierndeGuetermenge, min(MaximaleGueterherstellungErwerbstaetige, MaximaleGueterherstellungRohstoffe));
    Gueterherstellung = max(Gueterherstellung, 0);  
    
    % Berechnung der aktuellen Arbeitsplätze
    ArbeitsplaetzeUnternehmen = floor(Gueterherstellung / ProduktionProMitarbeiter)+1;
    
    % Berechnung der maximalen möglichen Entlassungen
    % Es können max. 20% der Mitarbeiter entlassen werden    
    if ArbeitsplaetzeUnternehmen < LetzteArbeitsplaetzeUnternehmen * (1-MaximaleEntlassungsrate)
        ArbeitsplaetzeUnternehmen = LetzteArbeitsplaetzeUnternehmen * (1-MaximaleEntlassungsrate);
        MaximaleGueterherstellungErwerbstaetige = ArbeitsplaetzeUnternehmen * ProduktionProMitarbeiter;
        Gueterherstellung = min(ProduzierndeGuetermenge, min(MaximaleGueterherstellungErwerbstaetige, MaximaleGueterherstellungRohstoffe));        
    end
    
    % Vergleich der Arbeitsnachfrage mit dem Arbeitsangebot
    ArbeitsangebotsNachfrageQuotient = ArbeitsplaetzeUnternehmen / Erwerbsfaehige;
    % Anpassung der Arbeitslöhne an das Angebot und die Nachfrage der
    % Arbeitsplaetze - max 3% Lohnsenkung oder Lohnsteigerung
    ArbeitsangebotsNachfrageQuotient= max(0.94,min(1.04,(ArbeitsangebotsNachfrageQuotient + 0.3)));
    Arbeitslohn = Arbeitslohn * ArbeitsangebotsNachfrageQuotient;
    
    % Berechnung der aktuell verbrauchten Ressourcen
    Rohstoffbestand = Rohstoffbestand - (floor(Gueterherstellung * RessourcenProGut)+1);
    
    % hergestellte Gütermenge
    Gueterbestand = Gueterbestand + Gueterherstellung;
    
    % Als Export-Angebot werden 30% der Güter vorgesehen
    GueterangebotAusland = Gueterbestand * 0.3;
    GueterangebotInland = Gueterbestand - GueterangebotAusland;          
    
    % Berechnung der Gehälter
    Gehaelter = ArbeitsplaetzeUnternehmen * Arbeitslohn;
    
    % Vorteil einer Investitionen-Rationalität berechnen
    InvestPruefungProduktionProMitarbeiter = (((1 + EffizienzsteigerungRationalitaet) ^ (TechnischeVerbesserungRationalitaet + 1)) * 2);
    InvestPruefungArbeitsplaetzeUnternehmen = floor(Gueterherstellung / InvestPruefungProduktionProMitarbeiter)+1;    
    InvesteinsparungRationalitaet = Arbeitslohn * (ArbeitsplaetzeUnternehmen - InvestPruefungArbeitsplaetzeUnternehmen);
    % Vorteil einer Investitionen-Ressourceneffizienz berechnen
    InvestPruefungRessourcenProGut = (1 / (1 + EffizienzsteigerungRessourcen)) ^ (TechnischeVerbesserungRessourcen + 1);
    InvestPruefungRessourcenbedarf = floor(Gueterherstellung * InvestPruefungRessourcenProGut)+1;    
    InvesteinsparungRessourcenbedarf = RessourcenAbgabeSteuersatz * ((Gueterherstellung * RessourcenProGut) - InvestPruefungRessourcenbedarf);    
    
    % Kosten für die nächste Investitionsstufe berechnen
    InvestkostenRationalitaet = Verbesserungskosten * (1 + Verbesserungskostensteigerung) ^ (TechnischeVerbesserungRationalitaet + 1);
    InvestkostenRessourcenEffizienz = Verbesserungskosten * (1 + Verbesserungskostensteigerung) ^ (TechnischeVerbesserungRessourcen + 1);
    
    % Prüfen, ob und welche Investition mehr Sinn macht
    % Das vorhandene Geld muss dabei doppelt so hoch sein, damit nicht mit
    % dem letzten Geld Investitionen durchgeführt werden
    Investition = 0;
    if (InvesteinsparungRationalitaet > InvesteinsparungRessourcenbedarf) && Geldbestand > InvestkostenRationalitaet*2 && InvesteinsparungRationalitaet > 0
        % Verbesserung Rationalität
        TechnischeVerbesserungRationalitaet = TechnischeVerbesserungRationalitaet + 1;
        Investition = InvestkostenRationalitaet;
        % Anstieg des Arbeitslohn auf Grund der Rationalitätsgewinne 
        Arbeitslohn = Arbeitslohn * (1 + Gehaltssteigerung);
    elseif Geldbestand > InvestkostenRessourcenEffizienz*2 && InvesteinsparungRessourcenbedarf > 0;
        % Verbesserung Ressourceneffizienz
        TechnischeVerbesserungRessourcen = TechnischeVerbesserungRessourcen + 1;
        Investition = InvestkostenRessourcenEffizienz;
    end
    
    % Ausgaben berechnen
    Ausgaben = RessourcenAbgabeSteuer + Gehaelter;
    
    % Der Preis der produzierten Warten richtet sich NICHT nach der Nachfrage 
    % und dem Angebot, sondern nach den Herrstellungskosten und dem 
    % angestrebten Gewinn. Welches ist der niedrigste Preis, damit das 
    % Unternehmen den angestrebten Gewinn erwirtschaftet und Investieren
    % kann
    Herstellkosten = Ausgaben / Gueterherstellung;
    % Es gibt eine maximale Preisteigerung welche durchgesetzt werden kann
    MaximalerGueterpreis = (1 + MaximalePreissteierung) * Gueterpreis;
    Gueterpreis = min(MaximalerGueterpreis, Herstellkosten * (1 + AngestrebterGewinn));   
    
    % Berechnung der Inflation
    Inflation = (InflationAlt + (Gueterpreis / AlterGueterpreis) - 1) / 2;
    InflationAlt = Inflation;
                
    % Gewinnberechnung
    Gewinn = Einnahmen - Ausgaben;            
    
    if Gewinn > 0
        % Anstieg des Arbeitslohn auf Grund der Gewinnsteigerung               
        Arbeitslohn = Arbeitslohn * (1 + Gehaltssteigerung);  
        
        % Steuerberechnung vom Gewinn
        SteuernUnternehmen = Gewinn * Steuersatz;
    else
        SteuernUnternehmen = 0;
    end

    Geldbestand = Geldbestand + Gewinn - (SteuernUnternehmen + Investition);
       
    % Wenn notwendig, neuen Kredit beantragen
    if Geldbestand < GewuenschterGeldbestand                
        % Kreditbedarf berechnen
        Kreditbedarf = GewuenschterGeldbestand - Geldbestand;
    else 
        Kreditbedarf = 0;
    end         
    
    % Kreditbedarf auf In- und Ausland aufteilen
    % Der Kredit mit dem geringeren Zinssatz wird bevorzugt und 70%
    % verwendet. Der teurere Kredit wird mit 30% verwendet.
    if KreditZinssatzInland <= KreditZinssatzAusland
        KreditbedarfInland = Kreditbedarf * 0.7;
        KreditbedarfAusland = Kreditbedarf * 0.3;
    else
        KreditbedarfAusland = Kreditbedarf * 0.7;
        KreditbedarfInland = Kreditbedarf * 0.3;        
    end

    % Berechnung der benötigten Ressourcen im nächsten Zeitabschnitt    
    Rohstoffbedarf = max(0, floor(Gueterherstellung * RessourcenProGut) + GewuenschterGuetervorrat - Rohstoffbestand);            
    
    % Auf Grund der Angebots-/Nachfragesituation kann der Güterpreis nicht
    % unter dem Arbeitslohn sein
    Gueterpreis = min(Gueterpreis, Arbeitslohn);
    % Wenn kein Konsum stattgefunden hat sinkt der Preis
    if GueterkonsumInland == 0
        Gueterpreis = Gueterpreis * (1-MaximalePreissteierung);
    end
    
    
    Wirtschaftswachstum = (Einnahmen / AlteEinnahmen) - 1;
    
    ArbeitslohnOut = Arbeitslohn;
    GueterpreisOut = Gueterpreis;
    TechnischeVerbesserungRationalitaetOut = TechnischeVerbesserungRationalitaet;
    TechnischeVerbesserungRessourcenOut = TechnischeVerbesserungRessourcen;
    LetzteArbeitsplaetzeUnternehmen = ArbeitsplaetzeUnternehmen;
